simulink model "Relaxation_Model"  (R2021b)
settings: Solver=ode4  StartTime=0.0  StopTime=0.01  FixedStep=1e-8
InitFcn:
  | params = [];
  | for ii=1:length(data.cnt)
  |     params = [params, [data.cnt(ii).params.model_coeff.value]'];
  | end
  | 
  | f_0 = 100000;
model workspace (MAT data in the model file):
  C_0 = 1
  ciao = 1
values from neighbouring files (symbols this model uses):
  data = struct()    [CreepAnalysis.m]    (also in CreepData.mat = ; FirstCreep.m; K0_comparison.mat = ; MisureRilassamento_cnt077145.mat = )
  ii = ii+1    (= 2)    [Creep_and_Tracking.m]    (also in Creep_and_Tracking_fit.m = find(x_long(ind)==x); FirstCreep.m = find(f>upper_bound | f<lower_bound); FromCreepToStatic.m = find(x_long(ind)==x); FromCreepToStatic_Times.m = find(x_long(ind)==x))
settings Model: Creator=stefa  LastModifiedBy=stefa
settings SolverCC: ShapePreserveControl=EnableAll

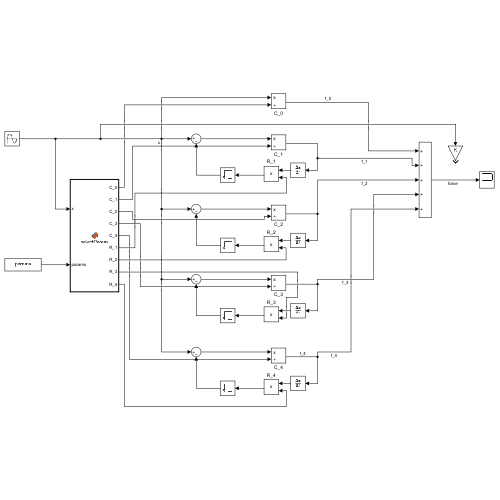
[thumbnail: Simulink's stored preview of the top-level diagram]
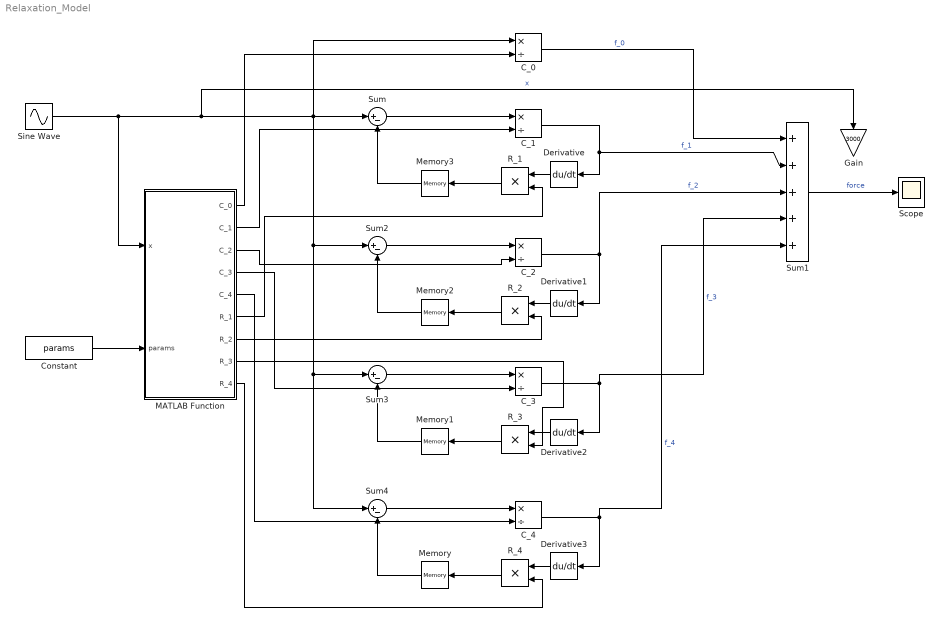
== system Relaxation_Model ==
  C_{0..4} (5 alike) : Product  Inputs=*/
  Constant : Constant  Value=params  VectorParams1D=off
  Derivative{,1..3} (4 alike) : Derivative
  Gain : Gain  Gain=3000
  MATLAB Function : MATLAB Function  TreatAsAtomicUnit=on
  Memory{,1..3} (4 alike) : Memory  InheritSampleTime=on  LinearizeMemory=on  LinearizeAsDelay=on
  R_{1..4} (4 alike) : Product
  Scope : Scope
  Sine Wave : Sin  Amplitude=0.01  Frequency=2*pi*100  SampleTime=0
  Sum{,2..4} (4 alike) : Sum  Inputs=|+-
  Sum1 : Sum  Inputs=+++++
  wires:
  Sum/1 -> C_1/1
  Derivative/1 -> R_1/1
  C_1/1 -> Derivative/1, Sum1/2  "f_1"
  C_0/1 -> Sum1/1  "f_0"
  Derivative1/1 -> R_2/1
  C_2/1 -> Sum1/3, Derivative1/1  "f_2"
  Sum2/1 -> C_2/1
  Sum3/1 -> C_3/1
  Derivative2/1 -> R_3/1
  Sine Wave/1 -> C_0/1, Sum4/1, Sum3/1, Sum2/1, Sum/1, Gain/1, MATLAB Function/1(x)  "x"
  C_3/1 -> Sum1/4, Derivative2/1  "f_3"
  Derivative3/1 -> R_4/1
  Sum4/1 -> C_4/1
  C_4/1 -> Sum1/5, Derivative3/1  "f_4"
  Sum1/1 -> Scope/1  "force"
  MATLAB Function/1(C_0) -> C_0/2
  MATLAB Function/2(C_1) -> C_1/2
  MATLAB Function/3(C_2) -> C_2/2
  MATLAB Function/4(C_3) -> C_3/2
  MATLAB Function/5(C_4) -> C_4/2
  MATLAB Function/6(R_1) -> R_1/2
  MATLAB Function/7(R_2) -> R_2/2
  MATLAB Function/8(R_3) -> R_3/2
  MATLAB Function/9(R_4) -> R_4/2
  Constant/1 -> MATLAB Function/2(params)
  R_1/1 -> Memory3/1
  R_2/1 -> Memory2/1
  R_3/1 -> Memory1/1
  R_4/1 -> Memory/1
  Memory3/1 -> Sum/2
  Memory2/1 -> Sum2/2
  Memory1/1 -> Sum3/2
  Memory/1 -> Sum4/2

== matlab function Relaxation_Model/MATLAB Function ==
  data: x input; C_0 output; C_1 output; C_2 output; C_3 output; C_4 output; R_1 output; R_2 output; R_3 output; R_4 output; params input
function [C_0, C_1, C_2, C_3, C_4, R_1, R_2, R_3, R_4] = selectParam(x, params)

% displ = params(1,:);
% % idx_max = min(find(x<displ));
% % idx_min = max(find(x>displ));
% idx_up = find(displ > x, 1, "first");
% idx_dw = find(displ < x, 1, "last");


C_0 = interp1(params(1,:), params(2,:), x);
C_1 = interp1(params(1,:), params(3,:), x);
C_2 = interp1(params(1,:), params(4,:), x);
C_3 = interp1(params(1,:), params(5,:), x);
C_4 = interp1(params(1,:), params(6,:), x);

R_1 = interp1(params(1,:), params(7,:), x);
R_2 = interp1(params(1,:), params(8,:), x);
R_3 = interp1(params(1,:), params(9,:), x);
R_4 = interp1(params(1,:), params(10,:), x);
